simulink model "d_analog_eq"  (R2019b)
settings: Solver=VariableStepAuto  StartTime=0.0  StopTime=10.0  MaxStep=0.00001  RelTol=1e-3
values from neighbouring files (symbols this model uses):
  Kd = 1/(exp(T0/Kda)-1)    [diffcode.m]
  Kda = T1    (= 0.1)    [diffcode.m]
  Kp = Kpa    (= 1)    [diffcode.m]
  Kpa = 1/(2*Tu*K1*K2)    [diffcode.m]
  st = 1    [diffcode.m]
  T0 = 0.001    [diffcode.m]
  T1 = 1 + 0.1*(2*rand()-1)    [diffcode.m]
  Tur = T0/2    (= 0.0005)    [diffcode.m]
settings Model: Creator=bedla  LastModifiedBy=bedla
settings DataIOCC: ReturnWorkspaceOutputs=off

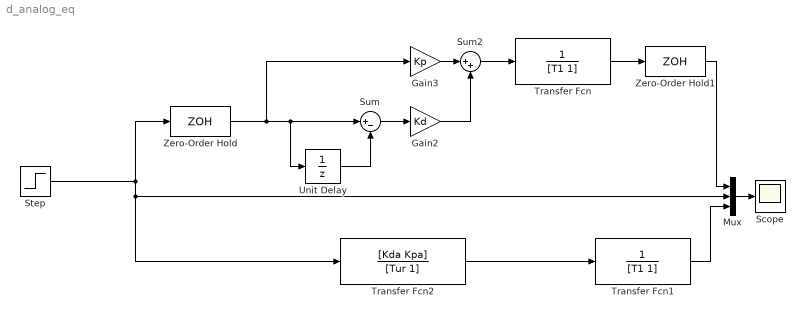
== system d_analog_eq ==
  Gain2 : Gain  Gain=Kd
  Gain3 : Gain  Gain=Kp
  Mux : Mux  Inputs=3
  Scope : Scope
  Step : Step  After=st  SampleTime=0
  Sum : Sum  Inputs=|+-
  Sum2 : Sum  Inputs=|++
  Transfer Fcn : TransferFcn  Denominator=[T1 1]
  Transfer Fcn1 : TransferFcn  Denominator=[T1 1]
  Transfer Fcn2 : TransferFcn  Numerator=[Kda Kpa]  Denominator=[Tur 1]
  Unit Delay : UnitDelay  SampleTime=T0  HasFrameUpgradeWarning=on
  Zero-Order Hold : ZeroOrderHold  SampleTime=T0
  Zero-Order Hold1 : ZeroOrderHold  SampleTime=T0
  wires:
  Step/1 -> Transfer Fcn2/1, Mux/2, Zero-Order Hold/1
  Transfer Fcn2/1 -> Transfer Fcn1/1
  Gain2/1 -> Sum2/2
  Zero-Order Hold/1 -> Gain3/1, Sum/1, Unit Delay/1
  Sum/1 -> Gain2/1
  Unit Delay/1 -> Sum/2
  Gain3/1 -> Sum2/1
  Sum2/1 -> Transfer Fcn/1
  Mux/1 -> Scope/1
  Transfer Fcn/1 -> Zero-Order Hold1/1
  Transfer Fcn1/1 -> Mux/3
  Zero-Order Hold1/1 -> Mux/1
